simulink model "mytest"  (R2018b)
settings: Solver=FixedStepAuto  StartTime=0.0  StopTime=50  FixedStep=0.001  RelTol=1e-3
undefined symbols (not defined in the file): wt
settings Model: Creator=chengqian  LastModifiedBy=chengqian

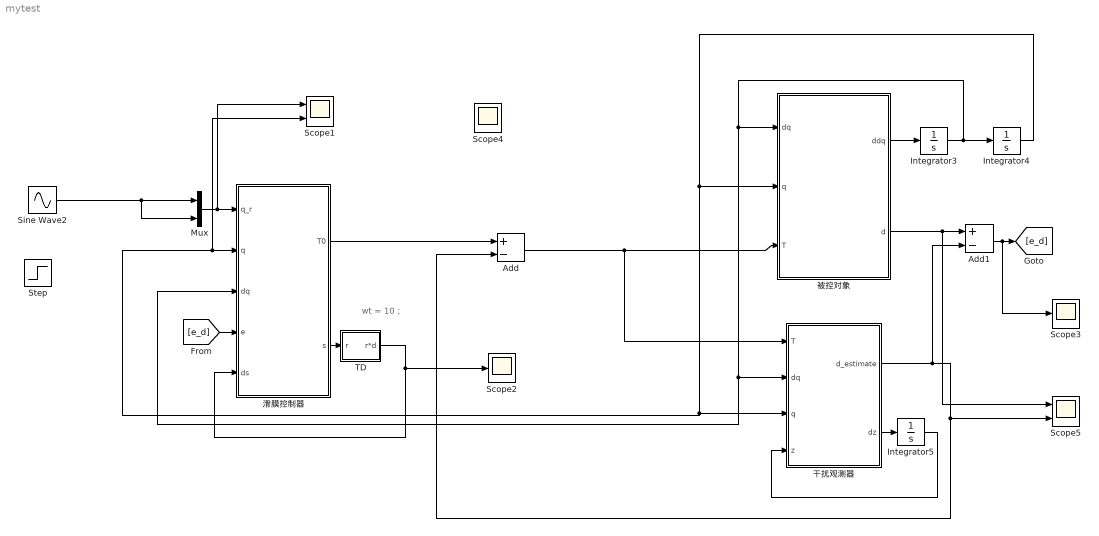
== system mytest ==
  note: wt = 10；
  Add : Sum  Inputs=+-
  Add1 : Sum  Inputs=+-
  Integrator3 : Integrator
  Integrator4 : Integrator
  Integrator5 : Integrator
  Mux : Mux  Inputs=2
  Scope1 : Scope  NumInputPorts=2
  Scope2 : Scope
  Scope3 : Scope
  Scope4 : Scope
  Scope5 : Scope  NumInputPorts=2
  Sine Wave2 : Sin  Frequency=2  SampleTime=0
  Step : Step  SampleTime=0
  TD : Subsystem
  干扰观测器 : MATLAB Function  TreatAsAtomicUnit=on
  滑膜控制器 : MATLAB Function  TreatAsAtomicUnit=on
  被控对象 : MATLAB Function  TreatAsAtomicUnit=on
  wires:
  被控对象/2(d) -> Scope5/1, Add1/1
  干扰观测器/2(dz) -> Integrator5/1
  [e_d] -> 滑膜控制器/4(e)
  滑膜控制器/2(s) -> TD/1(r)
  Sine Wave2/1 -> Mux/2, Mux/1
  Add1/1 -> Scope3/1, [e_d]
  Integrator3/1 -> 被控对象/1(dq), 滑膜控制器/3(dq), 干扰观测器/2(dq), Integrator4/1
  Integrator5/1 -> 干扰观测器/4(z)
  Integrator4/1 -> Scope1/2, 滑膜控制器/2(q), 干扰观测器/3(q), 被控对象/2(q)
  被控对象/1(ddq) -> Integrator3/1
  Mux/1 -> Scope1/1, 滑膜控制器/1(q_r)
  TD/1(r*d) -> Scope2/1, 滑膜控制器/5(ds)
  滑膜控制器/1(T0) -> Add/1
  干扰观测器/1(d_estimate) -> Scope5/2, Add/2, Add1/2
  Add/1 -> 被控对象/3(T), 干扰观测器/1(T)

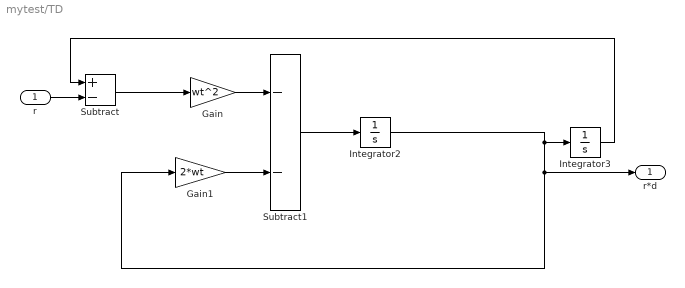
== system mytest/TD ==
  r : Inport
  Gain : Gain  Gain=wt^2
  Gain1 : Gain  Gain=2*wt
  Integrator2 : Integrator
  Integrator3 : Integrator
  Subtract : Sum  Inputs=+-
  Subtract1 : Sum  Inputs=--
  r*d : Outport
  wires:
  Integrator2/1 -> Integrator3/1, Gain1/1, r*d/1
  Gain1/1 -> Subtract1/2
  Subtract/1 -> Gain/1
  Gain/1 -> Subtract1/1
  Integrator3/1 -> Subtract/1
  Subtract1/1 -> Integrator2/1
  r/1 -> Subtract/2

== matlab function mytest/干扰观测器 ==
  data: T input; dq input; d_estimate output size=2; q input; dz output size=2; z input
function [d_estimate,dz] = fcn(T,dq,q,z)
%#codegen
g = 9.8;
p1 = 0.29;
p2 = 0.076;
p3 = 0.087;
p4 = 0.304;
p5 = 0.087;

L = [1.5 0;0 1.5];
q1 = q(1);
q2 = q(2);
dq1 = dq(1);
dq2 = dq(2);

C = [-p3*dq2*sin(q2) -p3*(dq1+dq2)*sin(q2);p3*dq1*sin(q2) 0];
G = [p4*g*cos(q1)+p5*g*cos(q1+q2);p5*g*cos(q1+q2)];

p = 1.5*[dq1;(dq1+dq2)];
dz = -L*z + L*(C*dq + G - T - p);
d_estimate = z + p;

== matlab function mytest/被控对象 ==
  data: dq input; q input; ddq output size=2; T input; d output size=2
function [ddq,d] = fcn(dq,q,T)
%#codegen
g = 9.8;
p1 = 0.29;
p2 = 0.076;
p3 = 0.087;
p4 = 0.304;
p5 = 0.087;

q1 = q(1);
q2 = q(2);

dq1 = dq(1);
dq2 = dq(2);
dq = [dq1;dq2];
M = [p1+p2+2*p3*cos(q2) p2+p3*cos(q2);p2+p3*cos(q2) p2];
C = [-p3*dq2*sin(q2) -p3*(dq1+dq2)*sin(q2);p3*dq1*sin(q2) 0];
G = [p4*g*cos(q1)+p5*g*cos(q1+q2);p5*g*cos(q1+q2)];

d = 0.5*sign(dq)+0.1*dq;%%随机扰动

ddq = inv(M)*(T+d-C*dq-G);

== matlab function mytest/滑膜控制器 ==
  data: q_r input; q input; dq input; T0 output size=2; e input; s output size=2; ds input
function [T0,s] = fcn(q_r,q,dq,e,ds)
%#codegen
r = 0.01;%%哪里是
namuta = 0.01;
g = 9.8;
p1 = 0.29;
p2 = 0.076;
p3 = 0.087;
p4 = 0.304;
p5 = 0.087;

x1 = q_r - q;
x11 = x1(1);
x12 = x1(2);
x2 = -dq;

q1 = q(1);
q2 = q(2);
dq1 = dq(1);
dq2 = dq(2);
dq = [dq1;dq2];

M = [p1+p2+2*p3*cos(q2) p2+p3*cos(q2);p2+p3*cos(q2) p2];
M1 = [p1+p2+2*p3*cos(x12) p2+p3*cos(x12);p2+p3*cos(x12) p2];
C = [-p3*dq2*sin(q2) -p3*(dq1+dq2)*sin(q2);p3*dq1*sin(q2) 0];
G = [p4*g*cos(q1)+p5*g*cos(q1+q2);p5*g*cos(q1+q2)];

s = sign(x1 + r*x2)*((sqrt(namuta*(namuta + norm(x1 + r*x2)))) - namuta)/2 + r*x2;

% ds1 = ds(1);
% ds2 = ds(2);
% 
% A1 = (ds1 + s(1)*sign(s(1)))/(ds1 + s(1))*sign(s(1));
% A2 = (ds2 + s(2)*sign(s(2)))/(ds2 + s(2))*sign(s(2));
% A = -[A1;A2];
%A = (ds + a)/(ds + sqrt(s));

beta = 200;
A = -beta*sign(s);

T_BS = (C-(2*M)/(3*r))*dq+G-e;
T_Vss = -M1*A;
T0 = T_BS + T_Vss;
